simulink model "sf_for"  (Simulink 6.0)
settings: Solver=FixedStepDiscrete  StartTime=0.0  StopTime=10.0  FixedStep=.1  RelTol=1e-3
libraries: simulink x1
settings Model: CovMetricSettings=dcmtr  Creator=The MathWorks Inc.  LastModifiedBy=batserve  ExtModeAutoUpdateStatusClock=off
settings DataIOCC: SignalLoggingName=sigsOut
settings DebuggingCC: CheckExecutionContextPreStartOutputMsg=on  CheckExecutionContextRuntimeOutputMsg=on  SolverPrmCheckMsg=none
settings HardwareCC: TargetUnknown=on

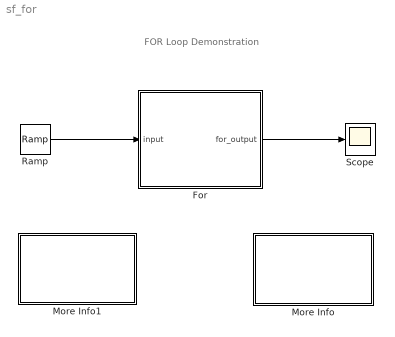
== system sf_for ==
  note: FOR Loop Demonstration
  For : Stateflow chart  PropExecContextAcrossSSBoundary=on
  More Info : Subsystem  PropExecContextAcrossSSBoundary=on
      mask Display: disp('Double click\nhere for\ninformation on\nthis demonstration')
  More Info1 : Subsystem  PropExecContextAcrossSSBoundary=on
      settings: OpenFcn=simcad(bdroot);
      mask Display: disp('Double click\nhere for\nSimulink\Stateflow\n Help')
  Ramp : simulink/Sources/Ramp  slope=1  start=0  X0=0
  Scope : Scope
      settings: TimeRange=10  YMin=0  YMax=2
  wires:
  Ramp/1 -> For/1(input)
  For/1(for_output) -> Scope/1

== system sf_for/More Info ==
  note: With the use of flow charts, Stateflow allows you to create C-Code or M-Code statements such as
      | the FOR loops. This particular demo shows how you can create a simple FOR Loop in Stateflow
      | using an input from Simulink. The equivalent statement in MATLAB is as follows:
      |
      | for i=1:20
      |    for_output = input(i)
      | end
      | for_output = 0;
      |
      | where INPUT is a ramp input with a slope of  1 simulated for 10 seconds. Notice how the
      | final_output is set to 0 after the FOR loops is exited. This is also apparent in the Scope from the
      | Simulink model.
  note: IF Statement

== system sf_for/More Info1 ==

== stateflow chart For ==
  note: Equivalent M-Code:
      |
      | for i=1:20
      |    for_output = input(i)
      | end
      | for_output = 0;
  (junction 4) -> (junction 6) : {for_output=0;}
  (default) -> (junction 4)
  (junction 4) -> (junction 5) : [i<20]
      | {for_output=input;i++;}
  data: input input double; for_output output double; i local double
